simulink model "EngPrt_PrtLimOvht1"  (R2016b)
settings: configuration reference "CodeGenConfigSet" (kept outside this file)
values from neighbouring files (symbols this model uses):
  EngPrt_facOvhtPrvAdd_CUR = Calibration.Parameter    [init_EngPrt_PrtLimOvht.m]    (also in init_EngPrt_PrtLimOvht_SIL.m = Simulink.Parameter)
  EngPrt_facOvhtPrvAdd_CURX = Calibration.Parameter    [init_EngPrt_PrtLimOvht.m]    (also in init_EngPrt_PrtLimOvht_SIL.m = Simulink.Parameter)
  EngPrt_facOvhtPrvCT_CUR = Calibration.Parameter    [init_EngPrt_PrtLimOvht.m]    (also in init_EngPrt_PrtLimOvht_SIL.m = Simulink.Parameter)
  EngPrt_facOvhtPrvCT_CURX = Calibration.Parameter    [init_EngPrt_PrtLimOvht.m]    (also in init_EngPrt_PrtLimOvht_SIL.m = Simulink.Parameter)
  EngPrt_facOvhtPrvDown_C = Calibration.Parameter    [init_EngPrt_PrtLimOvht.m]    (also in init_EngPrt_PrtLimOvht_SIL.m = Simulink.Parameter)
  EngPrt_facOvhtPrvFT_CUR = Calibration.Parameter    [init_EngPrt_PrtLimOvht.m]    (also in init_EngPrt_PrtLimOvht_SIL.m = Simulink.Parameter)
  EngPrt_facOvhtPrvFT_CURX = Calibration.Parameter    [init_EngPrt_PrtLimOvht.m]    (also in init_EngPrt_PrtLimOvht_SIL.m = Simulink.Parameter)
  EngPrt_facOvhtPrvIAT_CUR = Calibration.Parameter    [init_EngPrt_PrtLimOvht.m]    (also in init_EngPrt_PrtLimOvht_SIL.m = Simulink.Parameter)
  EngPrt_facOvhtPrvIAT_CURX = Calibration.Parameter    [init_EngPrt_PrtLimOvht.m]    (also in init_EngPrt_PrtLimOvht_SIL.m = Simulink.Parameter)
  EngPrt_facOvhtPrvIATCor_C = Calibration.Parameter    [init_EngPrt_PrtLimOvht.m]    (also in init_EngPrt_PrtLimOvht_SIL.m = Simulink.Parameter)
  EngPrt_facOvhtPrvOT_CUR = Calibration.Parameter    [init_EngPrt_PrtLimOvht.m]    (also in init_EngPrt_PrtLimOvht_SIL.m = Simulink.Parameter)
  EngPrt_facOvhtPrvOT_CURX = Calibration.Parameter    [init_EngPrt_PrtLimOvht.m]    (also in init_EngPrt_PrtLimOvht_SIL.m = Simulink.Parameter)
  EngPrt_facOvhtPrvUp_C = Calibration.Parameter    [init_EngPrt_PrtLimOvht.m]    (also in init_EngPrt_PrtLimOvht_SIL.m = Simulink.Parameter)
  EngPrt_numAir_C = Calibration.Parameter    [init_EngPrt_PrtLimOvht.m]    (also in init_EngPrt_PrtLimOvht_SIL.m = Simulink.Parameter)
  EngPrt_swtOvhtPrvDyn_C = Calibration.Parameter    [init_EngPrt_PrtLimOvht.m]    (also in init_EngPrt_PrtLimOvht_SIL.m = Simulink.Parameter)
  EngPrt_swtOvhtPrvOn_C = Calibration.Parameter    [init_EngPrt_PrtLimOvht.m]    (also in init_EngPrt_PrtLimOvht_SIL.m = Simulink.Parameter)
  EngPrt_tOvhtPrvAllwMax_C = Calibration.Parameter    [init_EngPrt_PrtLimOvht.m]    (also in init_EngPrt_PrtLimOvht_SIL.m = Simulink.Parameter)
  EngPrt_tOvhtPrvHighMapRef_C = Calibration.Parameter    [init_EngPrt_PrtLimOvht.m]    (also in init_EngPrt_PrtLimOvht_SIL.m = Simulink.Parameter)
  EngPrt_tOvhtPrvIATRef_CUR = Calibration.Parameter    [init_EngPrt_PrtLimOvht.m]    (also in init_EngPrt_PrtLimOvht_SIL.m = Simulink.Parameter)
  EngPrt_tOvhtPrvIATRef_CURX = Calibration.Parameter    [init_EngPrt_PrtLimOvht.m]    (also in init_EngPrt_PrtLimOvht_SIL.m = Simulink.Parameter)
  EngPrt_tOvhtPrvLowMapRef_C = Calibration.Parameter    [init_EngPrt_PrtLimOvht.m]    (also in init_EngPrt_PrtLimOvht_SIL.m = Simulink.Parameter)
  EngPrt_tOvhtPrvMinCalc_C = Calibration.Parameter    [init_EngPrt_PrtLimOvht.m]    (also in init_EngPrt_PrtLimOvht_SIL.m = Simulink.Parameter)
  EngPrt_trqOvhtPrvAdd_MAP = Calibration.Parameter    [init_EngPrt_PrtLimOvht.m]    (also in init_EngPrt_PrtLimOvht_SIL.m = Simulink.Parameter)
  EngPrt_trqOvhtPrvAdd_MAPX = Calibration.Parameter    [init_EngPrt_PrtLimOvht.m]    (also in init_EngPrt_PrtLimOvht_SIL.m = Simulink.Parameter)
  EngPrt_trqOvhtPrvAdd_MAPY = Calibration.Parameter    [init_EngPrt_PrtLimOvht.m]    (also in init_EngPrt_PrtLimOvht_SIL.m = Simulink.Parameter)
  EngPrt_trqOvhtPrvDynLimMax_C = Calibration.Parameter    [init_EngPrt_PrtLimOvht.m]    (also in init_EngPrt_PrtLimOvht_SIL.m = Simulink.Parameter)
  EngPrt_trqOvhtPrvDynLimMin_C = Calibration.Parameter    [init_EngPrt_PrtLimOvht.m]    (also in init_EngPrt_PrtLimOvht_SIL.m = Simulink.Parameter)
  EngPrt_trqOvhtPrvHigh_MAP = Calibration.Parameter    [init_EngPrt_PrtLimOvht.m]    (also in init_EngPrt_PrtLimOvht_SIL.m = Simulink.Parameter)
  EngPrt_trqOvhtPrvHigh_MAPX = Calibration.Parameter    [init_EngPrt_PrtLimOvht.m]    (also in init_EngPrt_PrtLimOvht_SIL.m = Simulink.Parameter)
  EngPrt_trqOvhtPrvHigh_MAPY = Calibration.Parameter    [init_EngPrt_PrtLimOvht.m]    (also in init_EngPrt_PrtLimOvht_SIL.m = Simulink.Parameter)
  EngPrt_trqOvhtPrvLow_MAP = Calibration.Parameter    [init_EngPrt_PrtLimOvht.m]    (also in init_EngPrt_PrtLimOvht_SIL.m = Simulink.Parameter)
  EngPrt_trqOvhtPrvLow_MAPX = Calibration.Parameter    [init_EngPrt_PrtLimOvht.m]    (also in init_EngPrt_PrtLimOvht_SIL.m = Simulink.Parameter)
  EngPrt_trqOvhtPrvLow_MAPY = Calibration.Parameter    [init_EngPrt_PrtLimOvht.m]    (also in init_EngPrt_PrtLimOvht_SIL.m = Simulink.Parameter)
  EngPrt_trqOvhtPrvMax_MAP = Calibration.Parameter    [init_EngPrt_PrtLimOvht.m]    (also in init_EngPrt_PrtLimOvht_SIL.m = Simulink.Parameter)
  EngPrt_trqOvhtPrvMax_MAPX = Calibration.Parameter    [init_EngPrt_PrtLimOvht.m]    (also in init_EngPrt_PrtLimOvht_SIL.m = Simulink.Parameter)
  EngPrt_trqOvhtPrvMax_MAPY = Calibration.Parameter    [init_EngPrt_PrtLimOvht.m]    (also in init_EngPrt_PrtLimOvht_SIL.m = Simulink.Parameter)
  EngPrt_trqOvhtPrvNRng_MAP = Calibration.Parameter    [init_EngPrt_PrtLimOvht.m]    (also in init_EngPrt_PrtLimOvht_SIL.m = Simulink.Parameter)
  EngPrt_trqOvhtPrvNRng_MAPX = Calibration.Parameter    [init_EngPrt_PrtLimOvht.m]    (also in init_EngPrt_PrtLimOvht_SIL.m = Simulink.Parameter)
  EngPrt_trqOvhtPrvNRng_MAPY = Calibration.Parameter    [init_EngPrt_PrtLimOvht.m]    (also in init_EngPrt_PrtLimOvht_SIL.m = Simulink.Parameter)
  EngPrt_trqOvhtPrvVRng_MAP = Calibration.Parameter    [init_EngPrt_PrtLimOvht.m]    (also in init_EngPrt_PrtLimOvht_SIL.m = Simulink.Parameter)
  EngPrt_trqOvhtPrvVRng_MAPX = Calibration.Parameter    [init_EngPrt_PrtLimOvht.m]    (also in init_EngPrt_PrtLimOvht_SIL.m = Simulink.Parameter)
  EngPrt_trqOvhtPrvVRng_MAPY = Calibration.Parameter    [init_EngPrt_PrtLimOvht.m]    (also in init_EngPrt_PrtLimOvht_SIL.m = Simulink.Parameter)
  TRQ_MAX = fi(1000,Trq_Nm)    [init_EngPrt_PrtLimOvht.m]    (also in init_EngPrt_PrtLimOvht_SIL.m)
undefined symbols (not defined in the file or in its folder): EngPrt_qOvhtPrvAdd_MAPX, EngPrt_qOvhtPrvHigh_MAPY, EngPrt_qOvhtPrvMax_MAPY, Switch_conv
libraries: CXLib x2
settings Model: Creator=Administrator  LastModifiedBy=zhoutinglin
settings ConfigSetRef: SourceLocation=Base Workspace

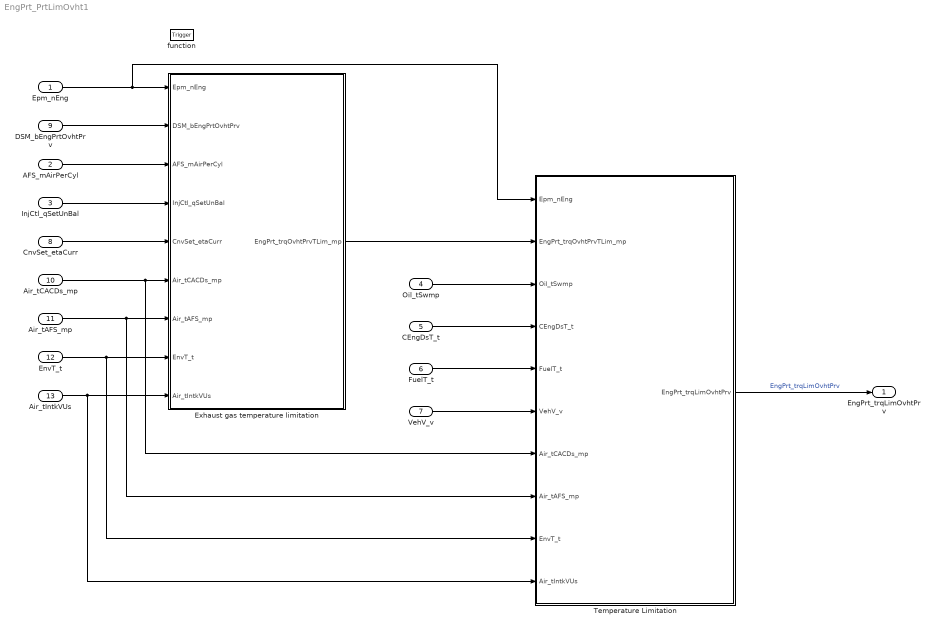
== system EngPrt_PrtLimOvht1 ==
  Epm_nEng : Inport  Tag=rpm  Description=Engine speed  OutMin=0  OutMax=6000  OutDataTypeStr=EngSpeed_rpm
  AFS_mAirPerCyl : Inport  Tag=mg/hub  Description=Air mass per cylinder  Port=2  OutMin=0  OutMax=16383  OutDataTypeStr=AirMass_mg_hub
  InjCtl_qSetUnBal : Inport  Tag=mg/hub  Description=Current injection quantity  Port=3  OutMin=-319  OutMax=319  OutDataTypeStr=FuelMass_mg_hub
  Oil_tSwmp : Inport  Tag=deg  Description=Oil temperature in oil sump  Port=4  OutMin=-50  OutMax=200  OutDataTypeStr=Temp_deg
  CEngDsT_t : Inport  Tag=deg  Description=engine coolant temperature after filter  Port=5  OutMin=-200  OutMax=200  OutDataTypeStr=Temp_deg
  FuelT_t : Inport  Tag=deg  Description=Temperature of fuel  Port=6  OutMin=-50  OutMax=150  OutDataTypeStr=Temp_deg
  VehV_v : Inport  Tag=km/h  Description=Vehicle speed  Port=7  OutMin=0  OutMax=250  OutDataTypeStr=VehSpeed_km_h
  CnvSet_etaCurr : Inport  Tag=Nm/(mg/hub)  Description=Current conversion efficiency  Port=8  OutMin=-255  OutMax=255  OutDataTypeStr=TrqEta_Nm_mg_hub
  DSM_bEngPrtOvhtPrv : Inport  Description=Status of FId_EngPrtOvhtPrv  Port=9  OutMin=0  OutMax=1  OutDataTypeStr=boolean
  Air_tCACDs_mp : Inport  Tag=deg  Description=Charge-air temperature downstream from charge-air cooler  Port=10  OutMin=-200  OutMax=200  OutDataTypeStr=Temp_deg
  Air_tAFS_mp : Inport  Tag=deg  Description=Induction air temperature at the HFM  Port=11  OutMin=-200  OutMax=200  OutDataTypeStr=Temp_deg
  EnvT_t : Inport  Tag=deg  Description=Environmental temperature  Port=12  OutMin=-200  OutMax=200  OutDataTypeStr=Temp_deg
  Air_tIntkVUs : Inport  Tag=deg  Description=Intake air temperature upstream of the inlet valve  Port=13  OutMin=-200  OutMax=200  OutDataTypeStr=Temp_deg
  function : TriggerPort  TriggerType=function-call  VariantControl=Variant
  Exhaust gas temperature limitation : Subsystem
  Temperature Limitation : Subsystem
  EngPrt_trqLimOvhtPrv : Outport  Tag=Nm  Description=Torque limitation value for engine protection from overheating  OutMin=-3276.8  OutMax=3276.7  OutDataTypeStr=Trq_Nm
  wires:
  Temperature Limitation/1(EngPrt_trqLimOvhtPrv) -> EngPrt_trqLimOvhtPrv/1  "EngPrt_trqLimOvhtPrv"
  Epm_nEng/1 -> Exhaust gas temperature limitation/1(Epm_nEng), Temperature Limitation/1(Epm_nEng)
  AFS_mAirPerCyl/1 -> Exhaust gas temperature limitation/3(AFS_mAirPerCyl)
  InjCtl_qSetUnBal/1 -> Exhaust gas temperature limitation/4(InjCtl_qSetUnBal)
  Exhaust gas temperature limitation/1(EngPrt_trqOvhtPrvTLim_mp) -> Temperature Limitation/2(EngPrt_trqOvhtPrvTLim_mp)
  Oil_tSwmp/1 -> Temperature Limitation/3(Oil_tSwmp)
  CEngDsT_t/1 -> Temperature Limitation/4(CEngDsT_t)
  FuelT_t/1 -> Temperature Limitation/5(FuelT_t)
  VehV_v/1 -> Temperature Limitation/6(VehV_v)
  CnvSet_etaCurr/1 -> Exhaust gas temperature limitation/5(CnvSet_etaCurr)
  DSM_bEngPrtOvhtPrv/1 -> Exhaust gas temperature limitation/2(DSM_bEngPrtOvhtPrv)
  Air_tCACDs_mp/1 -> Temperature Limitation/7(Air_tCACDs_mp), Exhaust gas temperature limitation/6(Air_tCACDs_mp)
  Air_tAFS_mp/1 -> Temperature Limitation/8(Air_tAFS_mp), Exhaust gas temperature limitation/7(Air_tAFS_mp)
  EnvT_t/1 -> Temperature Limitation/9(EnvT_t), Exhaust gas temperature limitation/8(EnvT_t)
  Air_tIntkVUs/1 -> Temperature Limitation/10(Air_tIntkVUs), Exhaust gas temperature limitation/9(Air_tIntkVUs)

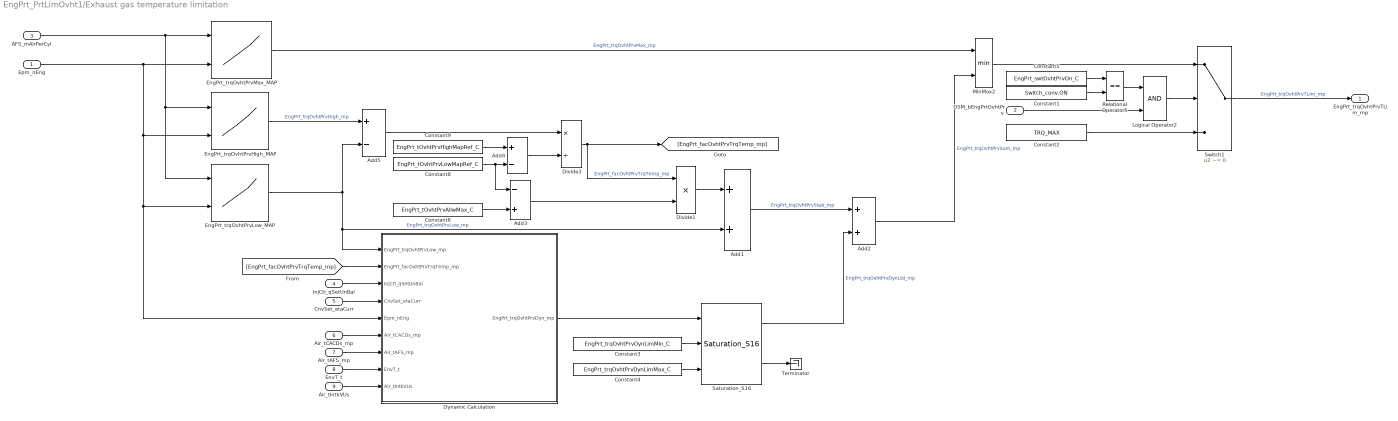
== system EngPrt_PrtLimOvht1/Exhaust gas temperature limitation ==
  Epm_nEng : Inport  Tag=rpm  Description=Average engine speed of one cylinder segment  OutMin=-12000  OutMax=12000  OutDataTypeStr=EngSpeed_rpm
  DSM_bEngPrtOvhtPrv : Inport  Description=Status of FId_EngPrtOvhtPrv  Port=2  OutMin=0  OutMax=1  OutDataTypeStr=boolean
  AFS_mAirPerCyl : Inport  Tag=mg/hub  Description=Filtered air mass per cylinder  Port=3  OutMin=0  OutMax=16383  OutDataTypeStr=AirMass_mg_hub
  InjCtl_qSetUnBal : Inport  Tag=mg/hub  Description=Current injection quantity  Port=4  OutMin=-319  OutMax=319  OutDataTypeStr=FuelMass_mg_hub
  CnvSet_etaCurr : Inport  Tag=Nm/(mg/hub)  Description=Current conversion efficiency  Port=5  OutMin=-255  OutMax=255  OutDataTypeStr=TrqEta_Nm_mg_hub
  Air_tCACDs_mp : Inport  Tag=deg  Description=Charge-air temperature downstream from charge-air cooler  Port=6  OutMin=-200  OutMax=200  OutDataTypeStr=Temp_deg
  Air_tAFS_mp : Inport  Tag=deg  Description=Induction air temperature at the HFM  Port=7  OutMin=-200  OutMax=200  OutDataTypeStr=Temp_deg
  EnvT_t : Inport  Tag=deg  Description=Environmental temperature  Port=8  OutMin=-200  OutMax=200  OutDataTypeStr=Temp_deg
  Air_tIntkVUs : Inport  Tag=deg  Description=Intake air temperature upstream of the inlet valve  Port=9  OutMin=-200  OutMax=200  OutDataTypeStr=Temp_deg
  Add1 : Sum  SaturateOnIntegerOverflow=on  InputSameDT=on
  Add2 : Sum  SaturateOnIntegerOverflow=on  InputSameDT=on
  Add3 : Sum  Inputs=-+  OutDataTypeStr=Temp_deg  RndMeth=Round  SaturateOnIntegerOverflow=on  InputSameDT=on
  Add4 : Sum  Inputs=+-  OutDataTypeStr=Temp_deg  RndMeth=Round  SaturateOnIntegerOverflow=on  InputSameDT=on
  Add5 : Sum  Inputs=+-  SaturateOnIntegerOverflow=on  InputSameDT=on
  Constant1 : Constant  Value=Switch_conv.ON  OutDataTypeStr=Inherit: Inherit via back propagation
  Constant2 : Constant  Value=TRQ_MAX
  Constant3 : Constant  Value=EngPrt_trqOvhtPrvDynLimMin_C
  Constant4 : Constant  Value=EngPrt_trqOvhtPrvDynLimMax_C
  Constant5 : Constant  Value=EngPrt_swtOvhtPrvOn_C
  Constant6 : Constant  Value=EngPrt_tOvhtPrvAllwMax_C
  Constant8 : Constant  Value=EngPrt_tOvhtPrvLowMapRef_C
  Constant9 : Constant  Value=EngPrt_tOvhtPrvHighMapRef_C
  Divide1 : Product  Inputs=**  OutDataTypeStr=Trq_Nm  SaturateOnIntegerOverflow=on
  Divide3 : Product  Inputs=*/  OutDataTypeStr=Inherit: Inherit via back propagation  RndMeth=Round  SaturateOnIntegerOverflow=on
  Dynamic Calculation : Subsystem
  EngPrt_trqOvhtPrvHigh_MAP : Lookup_n-D  BreakpointsForDimension1=EngPrt_trqOvhtPrvHigh_MAPY  BreakpointsForDimension2=EngPrt_trqOvhtPrvHigh_MAPX  IndexSearchMethod=Linear search  Table=EngPrt_trqOvhtPrvHigh_MAP  ExtrapMethod=Clip  InternalRulePriority=Speed  OutDataTypeStr=Inherit: Inherit via back propagation  RndMeth=Simplest  SaturateOnIntegerOverflow=on
  EngPrt_trqOvhtPrvLow_MAP : Lookup_n-D  BreakpointsForDimension1=EngPrt_trqOvhtPrvLow_MAPY  BreakpointsForDimension2=EngPrt_trqOvhtPrvLow_MAPX  IndexSearchMethod=Linear search  Table=EngPrt_trqOvhtPrvLow_MAP  ExtrapMethod=Clip  InternalRulePriority=Speed  OutDataTypeStr=Inherit: Inherit via back propagation  RndMeth=Simplest  SaturateOnIntegerOverflow=on
  EngPrt_trqOvhtPrvMax_MAP : Lookup_n-D  BreakpointsForDimension1=EngPrt_trqOvhtPrvMax_MAPY  BreakpointsForDimension2=EngPrt_trqOvhtPrvMax_MAPX  IndexSearchMethod=Linear search  Table=EngPrt_trqOvhtPrvMax_MAP  ExtrapMethod=Clip  InternalRulePriority=Speed  OutDataTypeStr=Inherit: Inherit via back propagation  RndMeth=Simplest  SaturateOnIntegerOverflow=on
  Logical Operator2 : Logic  OutDataTypeStr=boolean
  MinMax2 : MinMax  Inputs=2  SaturateOnIntegerOverflow=on  InputSameDT=on
  Relational Operator5 : RelationalOperator  Operator===  OutDataTypeStr=boolean  RndMeth=Simplest  InputSameDT=on
  Saturation_S16 : CXLib/Saturation_S16
  Switch1 : Switch  Criteria=u2 ~= 0  SaturateOnIntegerOverflow=on  InputSameDT=on
  Terminator : Terminator
  EngPrt_trqOvhtPrvTLim_mp : Outport
  wires:
  Logical Operator2/1 -> Switch1/2
  Constant5/1 -> Relational Operator5/1
  MinMax2/1 -> Switch1/1
  Switch1/1 -> EngPrt_trqOvhtPrvTLim_mp/1  "EngPrt_trqOvhtPrvTLim_mp"
  Add2/1 -> MinMax2/2  "EngPrt_trqOvhtPrvSum_mp"
  Saturation_S16/1 -> Add2/2  "EngPrt_trqOvhtPrvDynLtd_mp"
  Saturation_S16/2 -> Terminator/1
  Constant3/1 -> Saturation_S16/2
  Constant4/1 -> Saturation_S16/3
  Dynamic Calculation/1(EngPrt_trqOvhtPrvDyn_mp) -> Saturation_S16/1
  Add1/1 -> Add2/1  "EngPrt_trqOvhtPrvStab_mp"
  EngPrt_trqOvhtPrvLow_MAP/1 -> Add5/2, Dynamic Calculation/1(EngPrt_trqOvhtPrvLow_mp), Add1/2  "EngPrt_trqOvhtPrvLow_mp"
  Divide1/1 -> Add1/1
  Add3/1 -> Divide1/2
  Constant8/1 -> Add4/2, Add3/1
  Divide3/1 -> [EngPrt_facOvhtPrvTrqTemp_mp], Divide1/1  "EngPrt_facOvhtPrvTrqTemp_mp"
  Add4/1 -> Divide3/2
  Constant9/1 -> Add4/1
  Add5/1 -> Divide3/1
  EngPrt_trqOvhtPrvHigh_MAP/1 -> Add5/1  "EngPrt_trqOvhtPrvHigh_mp"
  EngPrt_trqOvhtPrvMax_MAP/1 -> MinMax2/1  "EngPrt_trqOvhtPrvMax_mp"
  AFS_mAirPerCyl/1 -> EngPrt_trqOvhtPrvLow_MAP/1, EngPrt_trqOvhtPrvHigh_MAP/1, EngPrt_trqOvhtPrvMax_MAP/1
  Epm_nEng/1 -> Dynamic Calculation/5(Epm_nEng), EngPrt_trqOvhtPrvLow_MAP/2, EngPrt_trqOvhtPrvHigh_MAP/2, EngPrt_trqOvhtPrvMax_MAP/2
  [EngPrt_facOvhtPrvTrqTemp_mp] -> Dynamic Calculation/2(EngPrt_facOvhtPrvTrqTemp_mp)
  InjCtl_qSetUnBal/1 -> Dynamic Calculation/3(InjCtl_qSetUnBal)
  Relational Operator5/1 -> Logical Operator2/1
  Constant2/1 -> Switch1/3
  DSM_bEngPrtOvhtPrv/1 -> Logical Operator2/2
  Constant1/1 -> Relational Operator5/2
  CnvSet_etaCurr/1 -> Dynamic Calculation/4(CnvSet_etaCurr)
  Constant6/1 -> Add3/2
  Air_tCACDs_mp/1 -> Dynamic Calculation/6(Air_tCACDs_mp)
  Air_tAFS_mp/1 -> Dynamic Calculation/7(Air_tAFS_mp)
  EnvT_t/1 -> Dynamic Calculation/8(EnvT_t)
  Air_tIntkVUs/1 -> Dynamic Calculation/9(Air_tIntkVUs)

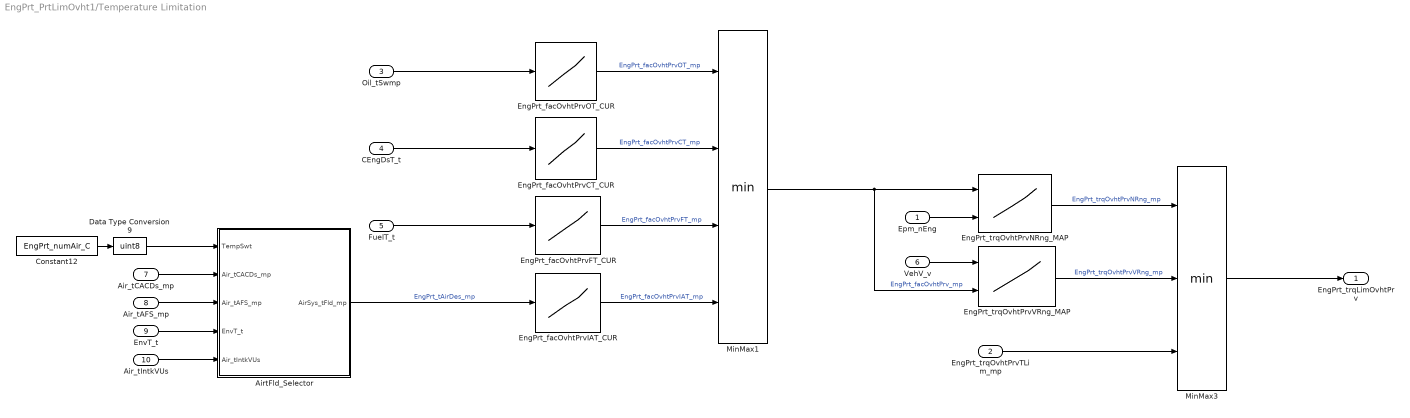
== system EngPrt_PrtLimOvht1/Temperature Limitation ==
  Epm_nEng : Inport  Tag=rpm  Description=Average engine speed of one cylinder segment  OutMin=-12000  OutMax=12000  OutDataTypeStr=EngSpeed_rpm
  EngPrt_trqOvhtPrvTLim_mp : Inport  Port=2
  Oil_tSwmp : Inport  Tag=deg  Description=engine oil temperature after filter  Port=3  OutMin=-50  OutMax=200  OutDataTypeStr=Temp_deg
  CEngDsT_t : Inport  Tag=deg  Description=engine coolant temperature after filter  Port=4  OutMin=-200  OutMax=200  OutDataTypeStr=Temp_deg
  FuelT_t : Inport  Tag=deg  Description=fuel temperature after filter  Port=5  OutMin=-50  OutMax=150  OutDataTypeStr=Temp_deg
  VehV_v : Inport  Tag=km/h  Description=Vehicle speed  Port=6  OutMin=0  OutMax=250  OutDataTypeStr=VehSpeed_km_h
  Air_tCACDs_mp : Inport  Tag=deg  Description=Charge-air temperature downstream from charge-air cooler  Port=7  OutMin=-200  OutMax=200  OutDataTypeStr=Temp_deg
  Air_tAFS_mp : Inport  Tag=deg  Description=Induction air temperature at the HFM  Port=8  OutMin=-200  OutMax=200  OutDataTypeStr=Temp_deg
  EnvT_t : Inport  Tag=deg  Description=Environmental temperature  Port=9  OutMin=-200  OutMax=200  OutDataTypeStr=Temp_deg
  Air_tIntkVUs : Inport  Tag=deg  Description=Intake air temperature upstream of the inlet valve  Port=10  OutMin=-200  OutMax=200  OutDataTypeStr=Temp_deg
  AirtFld_Selector : Subsystem
  Constant12 : Constant  Value=EngPrt_numAir_C  SampleTime=-1
  Data Type Conversion9 : DataTypeConversion  OutDataTypeStr=uint8
  EngPrt_facOvhtPrvCT_CUR : Lookup_n-D  NumberOfTableDimensions=1  BreakpointsForDimension1=EngPrt_facOvhtPrvCT_CURX  BreakpointsForDimension2=EngPrt_qOvhtPrvMax_MAPY  IndexSearchMethod=Linear search  Table=EngPrt_facOvhtPrvCT_CUR  ExtrapMethod=Clip  InternalRulePriority=Speed  OutDataTypeStr=Inherit: Inherit via back propagation  RndMeth=Simplest  SaturateOnIntegerOverflow=on
  EngPrt_facOvhtPrvFT_CUR : Lookup_n-D  NumberOfTableDimensions=1  BreakpointsForDimension1=EngPrt_facOvhtPrvFT_CURX  BreakpointsForDimension2=EngPrt_qOvhtPrvMax_MAPY  IndexSearchMethod=Linear search  Table=EngPrt_facOvhtPrvFT_CUR  ExtrapMethod=Clip  InternalRulePriority=Speed  OutDataTypeStr=Inherit: Inherit via back propagation  RndMeth=Simplest  SaturateOnIntegerOverflow=on
  EngPrt_facOvhtPrvIAT_CUR : Lookup_n-D  NumberOfTableDimensions=1  BreakpointsForDimension1=EngPrt_facOvhtPrvIAT_CURX  BreakpointsForDimension2=EngPrt_qOvhtPrvMax_MAPY  IndexSearchMethod=Linear search  Table=EngPrt_facOvhtPrvIAT_CUR  ExtrapMethod=Clip  InternalRulePriority=Speed  OutDataTypeStr=Inherit: Inherit via back propagation  RndMeth=Simplest  SaturateOnIntegerOverflow=on
  EngPrt_facOvhtPrvOT_CUR : Lookup_n-D  NumberOfTableDimensions=1  BreakpointsForDimension1=EngPrt_facOvhtPrvOT_CURX  BreakpointsForDimension2=EngPrt_qOvhtPrvMax_MAPY  IndexSearchMethod=Linear search  Table=EngPrt_facOvhtPrvOT_CUR  ExtrapMethod=Clip  InternalRulePriority=Speed  OutDataTypeStr=Inherit: Inherit via back propagation  RndMeth=Simplest  SaturateOnIntegerOverflow=on
  EngPrt_trqOvhtPrvNRng_MAP : Lookup_n-D  BreakpointsForDimension1=EngPrt_trqOvhtPrvNRng_MAPY  BreakpointsForDimension2=EngPrt_trqOvhtPrvNRng_MAPX  IndexSearchMethod=Linear search  Table=EngPrt_trqOvhtPrvNRng_MAP  ExtrapMethod=Clip  InternalRulePriority=Speed  OutDataTypeStr=Inherit: Inherit via back propagation  RndMeth=Simplest  SaturateOnIntegerOverflow=on
  EngPrt_trqOvhtPrvVRng_MAP : Lookup_n-D  BreakpointsForDimension1=EngPrt_trqOvhtPrvVRng_MAPY  BreakpointsForDimension2=EngPrt_trqOvhtPrvVRng_MAPX  IndexSearchMethod=Linear search  Table=EngPrt_trqOvhtPrvVRng_MAP  ExtrapMethod=Clip  InternalRulePriority=Speed  OutDataTypeStr=Inherit: Inherit via back propagation  RndMeth=Simplest  SaturateOnIntegerOverflow=on
  MinMax1 : MinMax  Inputs=4  SaturateOnIntegerOverflow=on  InputSameDT=on
  MinMax3 : MinMax  Inputs=3  SaturateOnIntegerOverflow=on  InputSameDT=on
  EngPrt_trqLimOvhtPrv : Outport  Tag=Nm  Description=Torque limitation due to high temperatures  OutMin=-3276.8  OutMax=3276.7  OutDataTypeStr=Trq_Nm
  wires:
  CEngDsT_t/1 -> EngPrt_facOvhtPrvCT_CUR/1
  EngPrt_trqOvhtPrvNRng_MAP/1 -> MinMax3/1  "EngPrt_trqOvhtPrvNRng_mp"
  Oil_tSwmp/1 -> EngPrt_facOvhtPrvOT_CUR/1
  FuelT_t/1 -> EngPrt_facOvhtPrvFT_CUR/1
  EngPrt_facOvhtPrvOT_CUR/1 -> MinMax1/1  "EngPrt_facOvhtPrvOT_mp"
  EngPrt_facOvhtPrvCT_CUR/1 -> MinMax1/2  "EngPrt_facOvhtPrvCT_mp"
  EngPrt_facOvhtPrvFT_CUR/1 -> MinMax1/3  "EngPrt_facOvhtPrvFT_mp"
  EngPrt_facOvhtPrvIAT_CUR/1 -> MinMax1/4  "EngPrt_facOvhtPrvIAT_mp"
  MinMax1/1 -> EngPrt_trqOvhtPrvVRng_MAP/2, EngPrt_trqOvhtPrvNRng_MAP/1  "EngPrt_facOvhtPrv_mp"
  Epm_nEng/1 -> EngPrt_trqOvhtPrvNRng_MAP/2
  VehV_v/1 -> EngPrt_trqOvhtPrvVRng_MAP/1
  EngPrt_trqOvhtPrvVRng_MAP/1 -> MinMax3/2  "EngPrt_trqOvhtPrvVRng_mp"
  EngPrt_trqOvhtPrvTLim_mp/1 -> MinMax3/3
  MinMax3/1 -> EngPrt_trqLimOvhtPrv/1
  Constant12/1 -> Data Type Conversion9/1
  AirtFld_Selector/1(AirSys_tFld_mp) -> EngPrt_facOvhtPrvIAT_CUR/1  "EngPrt_tAirDes_mp"
  Air_tCACDs_mp/1 -> AirtFld_Selector/2(Air_tCACDs_mp)
  Air_tAFS_mp/1 -> AirtFld_Selector/3(Air_tAFS_mp)
  EnvT_t/1 -> AirtFld_Selector/4(EnvT_t)
  Air_tIntkVUs/1 -> AirtFld_Selector/5(Air_tIntkVUs)
  Data Type Conversion9/1 -> AirtFld_Selector/1(TempSwt)

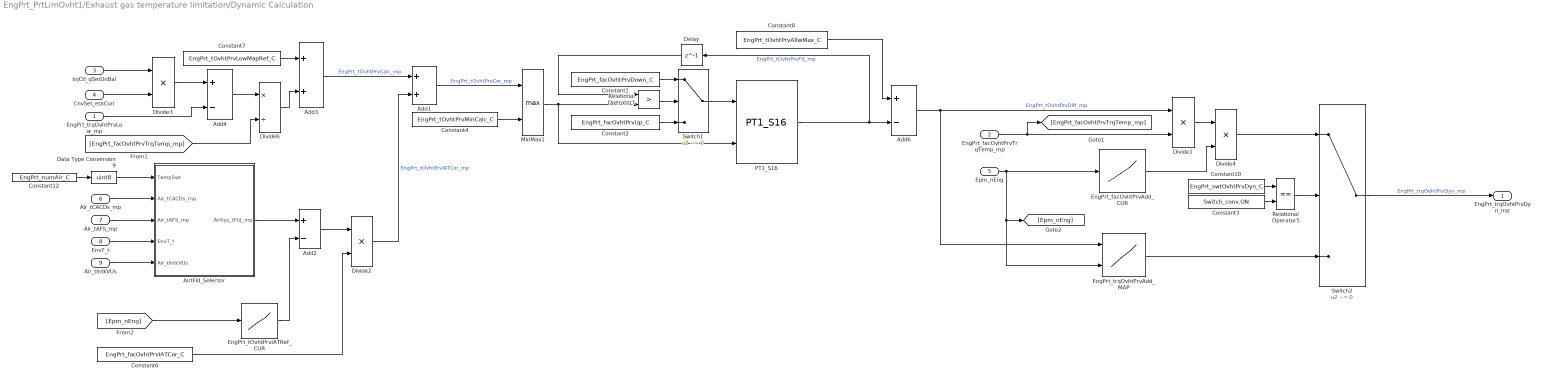
== system EngPrt_PrtLimOvht1/Exhaust gas temperature limitation/Dynamic Calculation ==
  EngPrt_trqOvhtPrvLow_mp : Inport
  EngPrt_facOvhtPrvTrqTemp_mp : Inport  Port=2
  InjCtl_qSetUnBal : Inport  Tag=mg/hub  Description=Current injection quantity  Port=3  OutMin=-319  OutMax=319  OutDataTypeStr=FuelMass_mg_hub
  CnvSet_etaCurr : Inport  Tag=Nm/(mg/hub)  Description=Current conversion efficiency  Port=4  OutMin=-255  OutMax=255  OutDataTypeStr=TrqEta_Nm_mg_hub
  Epm_nEng : Inport  Tag=rpm  Description=Average engine speed of one cylinder segment  Port=5  OutMin=-12000  OutMax=12000  OutDataTypeStr=EngSpeed_rpm
  Air_tCACDs_mp : Inport  Tag=deg  Description=Charge-air temperature downstream from charge-air cooler  Port=6  OutMin=-200  OutMax=200  OutDataTypeStr=Temp_deg
  Air_tAFS_mp : Inport  Tag=deg  Description=Induction air temperature at the HFM  Port=7  OutMin=-200  OutMax=200  OutDataTypeStr=Temp_deg
  EnvT_t : Inport  Tag=deg  Description=Environmental temperature  Port=8  OutMin=-200  OutMax=200  OutDataTypeStr=Temp_deg
  Air_tIntkVUs : Inport  Tag=deg  Description=Intake air temperature upstream of the inlet valve  Port=9  OutMin=-200  OutMax=200  OutDataTypeStr=Temp_deg
  Add1 : Sum  OutDataTypeStr=Inherit: Inherit via back propagation  SaturateOnIntegerOverflow=on  InputSameDT=on
  Add2 : Sum  Inputs=+-  OutDataTypeStr=Inherit: Inherit via back propagation  RndMeth=Round  SaturateOnIntegerOverflow=on  InputSameDT=on
  Add3 : Sum  OutDataTypeStr=Inherit: Inherit via back propagation  SaturateOnIntegerOverflow=on  InputSameDT=on
  Add4 : Sum  Inputs=+-  SaturateOnIntegerOverflow=on  InputSameDT=on
  Add6 : Sum  Inputs=+-  OutDataTypeStr=Inherit: Inherit via back propagation  SaturateOnIntegerOverflow=on  InputSameDT=on
  AirtFld_Selector : Subsystem
  Constant1 : Constant  Value=EngPrt_facOvhtPrvDown_C
  Constant10 : Constant  Value=EngPrt_swtOvhtPrvDyn_C
  Constant12 : Constant  Value=EngPrt_numAir_C  SampleTime=-1
  Constant2 : Constant  Value=EngPrt_facOvhtPrvUp_C
  Constant3 : Constant  Value=Switch_conv.ON  OutDataTypeStr=Inherit: Inherit via back propagation
  Constant4 : Constant  Value=EngPrt_tOvhtPrvMinCalc_C
  Constant6 : Constant  Value=EngPrt_facOvhtPrvIATCor_C
  Constant7 : Constant  Value=EngPrt_tOvhtPrvLowMapRef_C
  Constant8 : Constant  Value=EngPrt_tOvhtPrvAllwMax_C
  Data Type Conversion9 : DataTypeConversion  OutDataTypeStr=uint8
  Delay : Delay  DelayLength=1  InitialCondition=0
  Divide1 : Product  Inputs=**  OutDataTypeStr=Trq_Nm  RndMeth=Round  SaturateOnIntegerOverflow=on
  Divide2 : Product  Inputs=**  OutDataTypeStr=Temp_deg  SaturateOnIntegerOverflow=on
  Divide3 : Product  Inputs=**  OutDataTypeStr=Trq_Nm  SaturateOnIntegerOverflow=on
  Divide4 : Product  Inputs=**  OutDataTypeStr=Trq_Nm  RndMeth=Round  SaturateOnIntegerOverflow=on
  Divide6 : Product  Inputs=*/  OutDataTypeStr=Temp_deg  RndMeth=Round  SaturateOnIntegerOverflow=on
  EngPrt_facOvhtPrvAdd_CUR : Lookup_n-D  NumberOfTableDimensions=1  BreakpointsForDimension1=EngPrt_facOvhtPrvAdd_CURX  BreakpointsForDimension2=EngPrt_qOvhtPrvAdd_MAPX  IndexSearchMethod=Linear search  Table=EngPrt_facOvhtPrvAdd_CUR  ExtrapMethod=Clip  InternalRulePriority=Speed  OutDataTypeStr=Inherit: Inherit via back propagation  RndMeth=Simplest  SaturateOnIntegerOverflow=on
  EngPrt_tOvhtPrvIATRef_CUR : Lookup_n-D  NumberOfTableDimensions=1  BreakpointsForDimension1=EngPrt_tOvhtPrvIATRef_CURX  BreakpointsForDimension2=EngPrt_qOvhtPrvHigh_MAPY  IndexSearchMethod=Linear search  Table=EngPrt_tOvhtPrvIATRef_CUR  ExtrapMethod=Clip  InternalRulePriority=Speed  OutDataTypeStr=Inherit: Inherit via back propagation  RndMeth=Simplest  SaturateOnIntegerOverflow=on
  EngPrt_trqOvhtPrvAdd_MAP : Lookup_n-D  BreakpointsForDimension1=EngPrt_trqOvhtPrvAdd_MAPY  BreakpointsForDimension2=EngPrt_trqOvhtPrvAdd_MAPX  IndexSearchMethod=Linear search  Table=EngPrt_trqOvhtPrvAdd_MAP  ExtrapMethod=Clip  InternalRulePriority=Speed  OutDataTypeStr=Inherit: Inherit via back propagation  RndMeth=Simplest  SaturateOnIntegerOverflow=on
  MinMax1 : MinMax  Function=max  Inputs=2  SaturateOnIntegerOverflow=on  InputSameDT=on
  PT1_S16 : CXLib/PT1_S16
  Relational Operator1 : RelationalOperator  Operator=>  OutDataTypeStr=boolean  RndMeth=Nearest  InputSameDT=on
  Relational Operator5 : RelationalOperator  Operator===  OutDataTypeStr=boolean  RndMeth=Simplest  InputSameDT=on
  Switch1 : Switch  Criteria=u2 ~= 0  SaturateOnIntegerOverflow=on  InputSameDT=on
  Switch2 : Switch  Criteria=u2 ~= 0  SaturateOnIntegerOverflow=on  InputSameDT=on
  EngPrt_trqOvhtPrvDyn_mp : Outport
  wires:
  Switch2/1 -> EngPrt_trqOvhtPrvDyn_mp/1  "EngPrt_trqOvhtPrvDyn_mp"
  Constant10/1 -> Relational Operator5/1
  EngPrt_facOvhtPrvAdd_CUR/1 -> Divide4/2
  Epm_nEng/1 -> EngPrt_trqOvhtPrvAdd_MAP/2, [Epm_nEng], EngPrt_facOvhtPrvAdd_CUR/1
  Divide1/1 -> Divide4/1
  EngPrt_facOvhtPrvTrqTemp_mp/1 -> [EngPrt_facOvhtPrvTrqTemp_mp], Divide1/2
  EngPrt_trqOvhtPrvAdd_MAP/1 -> Switch2/3
  Add6/1 -> EngPrt_trqOvhtPrvAdd_MAP/1, Divide1/1  "EngPrt_tOvhtPrvDiff_mp"
  Constant8/1 -> Add6/1
  Constant2/1 -> Switch1/3
  Constant1/1 -> Switch1/1
  Relational Operator1/1 -> Switch1/2
  Delay/1 -> Relational Operator1/1
  Constant4/1 -> MinMax1/2
  Add1/1 -> MinMax1/1  "EngPrt_tOvhtPrvCor_mp"
  Divide2/1 -> Add1/2  "EngPrt_tOvhtPrvIATCor_mp"
  Constant6/1 -> Divide2/2
  Add2/1 -> Divide2/1
  EngPrt_tOvhtPrvIATRef_CUR/1 -> Add2/2
  Add3/1 -> Add1/1  "EngPrt_tOvhtPrvCalc_mp"
  Add4/1 -> Divide6/1
  EngPrt_trqOvhtPrvLow_mp/1 -> Add4/2
  InjCtl_qSetUnBal/1 -> Divide3/1
  Divide6/1 -> Add3/2
  Constant7/1 -> Add3/1
  [EngPrt_facOvhtPrvTrqTemp_mp] -> Divide6/2
  [Epm_nEng] -> EngPrt_tOvhtPrvIATRef_CUR/1
  Divide4/1 -> Switch2/1
  Switch1/1 -> PT1_S16/1
  MinMax1/1 -> PT1_S16/2, Relational Operator1/2
  PT1_S16/1 -> Delay/1, Add6/2  "EngPrt_tOvhtPrvFlt_mp"
  Relational Operator5/1 -> Switch2/2
  Constant3/1 -> Relational Operator5/2
  AirtFld_Selector/1(AirSys_tFld_mp) -> Add2/1
  CnvSet_etaCurr/1 -> Divide3/2
  Divide3/1 -> Add4/1
  Data Type Conversion9/1 -> AirtFld_Selector/1(TempSwt)
  Air_tCACDs_mp/1 -> AirtFld_Selector/2(Air_tCACDs_mp)
  Air_tAFS_mp/1 -> AirtFld_Selector/3(Air_tAFS_mp)
  EnvT_t/1 -> AirtFld_Selector/4(EnvT_t)
  Air_tIntkVUs/1 -> AirtFld_Selector/5(Air_tIntkVUs)
  Constant12/1 -> Data Type Conversion9/1

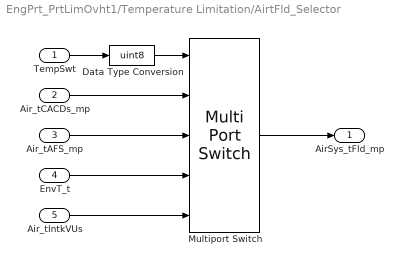
== system EngPrt_PrtLimOvht1/Temperature Limitation/AirtFld_Selector ==
  TempSwt : Inport
  Air_tCACDs_mp : Inport  Tag=deg  Description=Charge-air temperature downstream from charge-air cooler  Port=2
  Air_tAFS_mp : Inport  Tag=deg  Description=Induction air temperature at the HFM  Port=3
  EnvT_t : Inport  Tag=deg  Description=Environmental temperature  Port=4
  Air_tIntkVUs : Inport  Tag=deg  Description=Intake air temperature upstream of the inlet valve  Port=5
  Data Type Conversion : DataTypeConversion  OutDataTypeStr=uint8
  Multiport Switch : MultiPortSwitch  DataPortOrder=Zero-based contiguous  Inputs=4
  AirSys_tFld_mp : Outport  Tag=deg  Description=Engine temperature field
  wires:
  Air_tCACDs_mp/1 -> Multiport Switch/2
  Multiport Switch/1 -> AirSys_tFld_mp/1
  EnvT_t/1 -> Multiport Switch/4
  Air_tAFS_mp/1 -> Multiport Switch/3
  Data Type Conversion/1 -> Multiport Switch/1
  TempSwt/1 -> Data Type Conversion/1
  Air_tIntkVUs/1 -> Multiport Switch/5

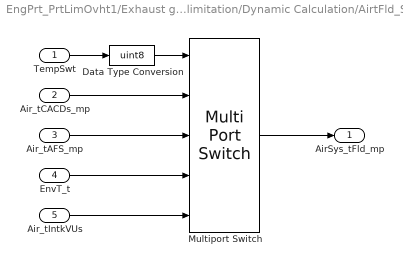
== system EngPrt_PrtLimOvht1/Exhaust gas temperature limitation/Dynamic Calculation/AirtFld_Selector ==
  TempSwt : Inport
  Air_tCACDs_mp : Inport  Tag=deg  Description=Charge-air temperature downstream from charge-air cooler  Port=2
  Air_tAFS_mp : Inport  Tag=deg  Description=Induction air temperature at the HFM  Port=3
  EnvT_t : Inport  Tag=deg  Description=Environmental temperature  Port=4
  Air_tIntkVUs : Inport  Tag=deg  Description=Intake air temperature upstream of the inlet valve  Port=5
  Data Type Conversion : DataTypeConversion  OutDataTypeStr=uint8
  Multiport Switch : MultiPortSwitch  DataPortOrder=Zero-based contiguous  Inputs=4
  AirSys_tFld_mp : Outport  Tag=deg  Description=Engine temperature field
  wires:
  Air_tCACDs_mp/1 -> Multiport Switch/2
  Multiport Switch/1 -> AirSys_tFld_mp/1
  EnvT_t/1 -> Multiport Switch/4
  Air_tAFS_mp/1 -> Multiport Switch/3
  Data Type Conversion/1 -> Multiport Switch/1
  TempSwt/1 -> Data Type Conversion/1
  Air_tIntkVUs/1 -> Multiport Switch/5
